simulink model "main"  (Simulink 4.00)
settings: Solver=ode45  StartTime=0.0  StopTime=10.0  RelTol=1e-3
settings Model: LastModifiedBy=User

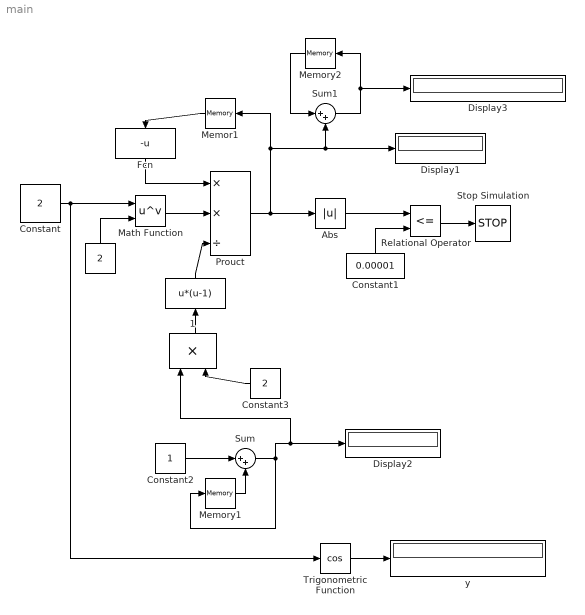
== system main ==
  " " : Constant  Orientation=up  Value=2
  "  " : Fcn  Orientation=up  Expr=u*(u-1)
  " 1" : Product  Orientation=up  Inputs=2  Multiplication=Element-wise(.*)  SaturateOnIntegerOverflow=on
  Abs : Abs  SaturateOnIntegerOverflow=on
  Constant : Constant  Value=2
  Constant1 : Constant  Orientation=up  Value=0.00001
  Constant2 : Constant  Value=1
  Constant3 : Constant  Orientation=left  Value=2
  Display1 : Display
      settings: Format=short
  Display2 : Display
      settings: Format=short
  Display3 : Display
  Fcn : Fcn  Orientation=down  Expr=-u
  Math Function : Math  Operator=pow  OutputSignalType=auto
  "Memor1 " : Memory  Orientation=left  X0=1  InheritSampleTime=off
      settings: RTWStateStorageClass=Auto
  Memory1 : Memory  X0=0  InheritSampleTime=off
      settings: RTWStateStorageClass=Auto
  Memory2 : Memory  Orientation=left  X0=1  InheritSampleTime=off
      settings: RTWStateStorageClass=Auto
  Prouct : Product  Inputs=**/  Multiplication=Element-wise(.*)  SaturateOnIntegerOverflow=off
  Relational Operator : RelationalOperator  Operator=<=
  Stop Simulation : Stop
  Sum : Sum  Inputs=|++  SaturateOnIntegerOverflow=on
  Sum1 : Sum  Inputs=|++  SaturateOnIntegerOverflow=off
  Trigonometric Function : Trigonometry  Operator=cos  OutputSignalType=auto
  y : Display
  wires:
  Trigonometric Function/1 -> y/1
  "Memor1 "/1 -> Fcn/1
  Prouct/1 -> "Memor1 "/1, Display1/1, Sum1/2, Abs/1
  Abs/1 -> Relational Operator/1
  Constant1/1 -> Relational Operator/2
  Relational Operator/1 -> Stop Simulation/1
  Constant2/1 -> Sum/1
  Memory1/1 -> Sum/2
  Sum1/1 -> Memory2/1, Display3/1
  Memory2/1 -> Sum1/1
  " "/1 -> Math Function/2
  Math Function/1 -> Prouct/2
  Fcn/1 -> Prouct/1
  "  "/1 -> Prouct/3
  " 1"/1 -> "  "/1
  Constant3/1 -> " 1"/2
  Constant/1 -> Math Function/1, Trigonometric Function/1
  Sum/1 -> Display2/1, " 1"/1, Memory1/1
